simulink model "simulink_to_mp"  (R2024b)
settings: Solver=VariableStepAuto  StartTime=0.0  StopTime=inf  RelTol=1e-3
undefined symbols (not defined in the file): Payload
libraries: uavmavlinklib x4, dspnetwork x2
settings Model: Creator=ercu  LastModifiedBy=ercu

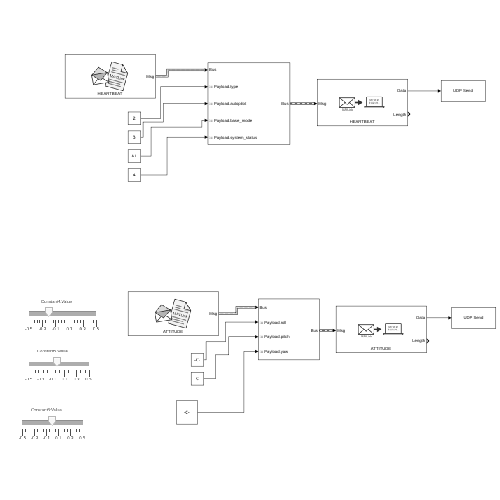
[thumbnail: Simulink's stored preview of the top-level diagram]
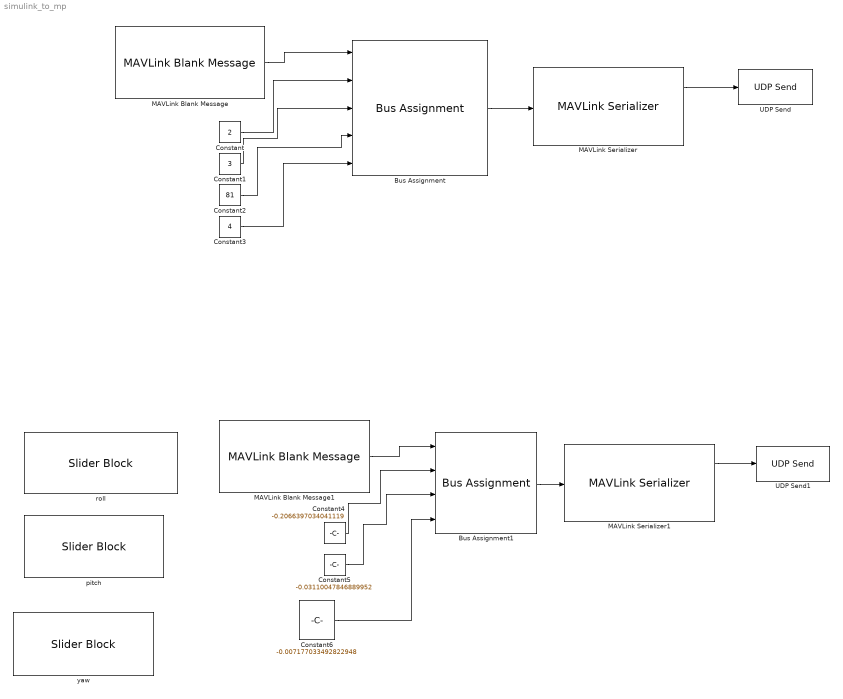
== system simulink_to_mp ==
  Bus Assignment : BusAssignment  AssignedSignals=Payload.type,Payload.autopilot,Payload.base_mode,Payload.system_status
  Bus Assignment1 : BusAssignment  AssignedSignals=Payload.roll,Payload.pitch,Payload.yaw
  Constant : Constant  Value=2  OutDataTypeStr=uint8
  Constant1 : Constant  Value=3  OutDataTypeStr=uint8
  Constant2 : Constant  Value=81  OutDataTypeStr=uint8
  Constant3 : Constant  Value=4  OutDataTypeStr=uint8
  Constant4 : Constant  Value=-0.2066397034041119  OutDataTypeStr=single
  Constant5 : Constant  Value=-0.03110047846889952  OutDataTypeStr=single
  Constant6 : Constant  Value=-0.007177033492822948  OutDataTypeStr=single
  MAVLink Blank Message : uavmavlinklib/MAVLink Blank Message  dialectSource=Select from standard MAVLink dialects  dialect=common.xml  dialectCustom=common.xml  version=2  messageType=HEARTBEAT  SystemID=1  ComponentID=1  SampleTime=inf
  MAVLink Blank Message1 : uavmavlinklib/MAVLink Blank Message  dialectSource=Select from standard MAVLink dialects  dialect=common.xml  dialectCustom=common.xml  version=2  messageType=ATTITUDE  SystemID=1  ComponentID=1  SampleTime=inf
  MAVLink Serializer : uavmavlinklib/MAVLink Serializer  dialectSource=Select from standard MAVLink dialects  dialect=common.xml  dialectCustom=common.xml  version=2  messageType=HEARTBEAT
  MAVLink Serializer1 : uavmavlinklib/MAVLink Serializer  dialectSource=Select from standard MAVLink dialects  dialect=common.xml  dialectCustom=common.xml  version=2  messageType=ATTITUDE
  UDP Send : dspnetwork/UDP Send  remoteURL='127.0.0.1'  remotePort=14550  localURL='0.0.0.0'  localPortSource=Automatically determine  localPort=-1  sendBufferSize=8192  sampletime=-1  blockPlatform=[]  separateLengthPort=0
      settings: LibrarySourceBlock=dspsnks4/UDP Send
  UDP Send1 : dspnetwork/UDP Send  remoteURL='127.0.0.1'  remotePort=14550  localURL='0.0.0.0'  localPortSource=Automatically determine  localPort=-1  sendBufferSize=8192  sampletime=-1  blockPlatform=[]  separateLengthPort=0
      settings: LibrarySourceBlock=dspsnks4/UDP Send
  pitch : SliderBlock  ScaleMin=-0.5  ScaleMax=0.5
  roll : SliderBlock  ScaleMin=-0.5  ScaleMax=0.5
  yaw : SliderBlock  ScaleMin=-0.5  ScaleMax=0.5
  wires:
  MAVLink Blank Message/1 -> Bus Assignment/1
  Bus Assignment/1 -> MAVLink Serializer/1
  Constant/1 -> Bus Assignment/2
  Constant1/1 -> Bus Assignment/3
  Constant2/1 -> Bus Assignment/4
  Constant3/1 -> Bus Assignment/5
  MAVLink Serializer/1 -> UDP Send/1
  MAVLink Blank Message1/1 -> Bus Assignment1/1
  Constant4/1 -> Bus Assignment1/2
  Constant5/1 -> Bus Assignment1/3
  Constant6/1 -> Bus Assignment1/4
  Bus Assignment1/1 -> MAVLink Serializer1/1
  MAVLink Serializer1/1 -> UDP Send1/1
